simulink model "PID"  (R2021a)
settings: Solver=VariableStepAuto  StartTime=0.0  StopTime=2  RelTol=1e-3
libraries: cstblocks x2
settings Model: Creator=User  LastModifiedBy=faust

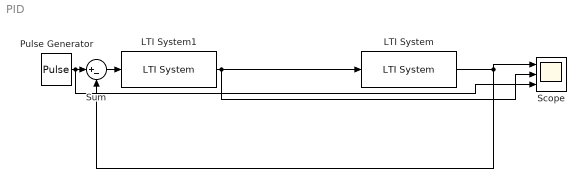
== system PID ==
  LTI System : cstblocks/LTI System  sys=P  IC=[]
  LTI System1 : cstblocks/LTI System  sys=C_dig  IC=[]
  Pulse Generator : DiscretePulseGenerator  PulseType=Time based  Amplitude=0.1  Period=1  PulseWidth=5
  Scope : Scope  NumInputPorts=3
  Sum : Sum  Inputs=|+-
  wires:
  Sum/1 -> LTI System1/1
  LTI System/1 -> Sum/2, Scope/1
  Pulse Generator/1 -> Scope/3, Sum/1
  LTI System1/1 -> LTI System/1, Scope/2
